simulink model "fusionAlg"  (R2018b)
settings: Solver=FixedStepDiscrete  StartTime=0.0  StopTime=inf  FixedStep=0.01  RelTol=1e-3
PostLoadFcn:
  | if any(exist('dsrtsu_mdlpostloadfcn', 'file') ~= 0), dsrtsu_mdlpostloadfcn('Execute', bdroot); end
model workspace (MAT data in the model file):
  cs : Simulink.ConfigSet (value not decoded)
(part 1 of 24)
settings Model: DSRTSU_INTERNAL_RTI_VER=540  DSRTSU_INTERNAL_RTI_TYPE=rti1401  RTICANMMDATA=struct('GeneralSetupData',struct('modelroot','F:\DatabaseZO\08.Code\Model\ZOP_Integration','generalsettings',struct('filesettings',struct('destfolder',struct('Name','RTICANMM_FILES','Check',1),'buildfolder',struct('Name','.','Check',1),'AbsDestfolder',struct('Name','F:\DatabaseZO\08.Code\Model\ZOP_Integration\RTICANMM_FILES'),'AbsBuildfolder',struct('Name','F:\DatabaseZO\08.Code\Model\ZOP_Integration'))),'options',struct('addpaths',1,'rmpaths',1,'addtrcexclusion',logical(1),'cannavigator',struct('checkmonitoring',0),'show_usrtrc',0,'use_usrtrc',0),'advanced',struct('options',ones(1,100)),'MPSetup',{{}},'RTI',struct('Type','RTI1401','Ver','7.12','Date','02-May-2019'),'modelname','fusionAlg','block','fusionAlg'))  DSRTSU_INTERNAL_RTIFPGA=130  Creator=One-J  LastModifiedBy=zjw
settings OptimizationCC: BlockReduction=off  ConditionallyExecuteInputs=off  DefaultUnderspecifiedDataType=single  BufferReuse=off  EnhancedBackFolding=on  ExpressionFolding=off  PassReuseOutputArgsThreshold=0  LocalBlockOutputs=off  OptimizeBlockOrder=speed  DifferentSizesBufferReuse=on
settings DebuggingCC: ParameterTunabilityLossMsg=error
settings HardwareCC: ProdBitPerPointer=32  ProdBitPerSizeT=32  ProdBitPerPtrDiffT=32  ProdLargestAtomicInteger=Integer  ProdEndianess=BigEndian  ProdWordSize=32  ProdHWDeviceType=Custom Processor->Custom  TargetIntDivRoundTo=Zero  TargetEndianess=BigEndian  TargetHWDeviceType=Custom Processor->Custom
settings ModelReferenceCC: ModelReferenceNumInstancesAllowed=Single
settings SFSimCC: MATLABDynamicMemAlloc=off
settings RTWCC: SystemTargetFile=rti1401.tlc  MakeCommand=make_rti  TemplateMakefile=rti1401.tmf  Description=dSPACE DS1401 Hardware Platform  GenerateReport=on  LaunchReport=on
settings CodeAppCC: OperatorAnnotations=on
settings STFCustomTargetCC: ParMdlRefBuildCompliant=on  SystemTargetFile=rti1401.tlc
settings GRTTargetCC: TargetLangStandard=C89/C90 (ANSI)  CompOptLevelCompliant=off  ConcurrentExecutionCompliant=off  CombineOutputUpdateFcns=off  MatFileLogging=off  CPPClassGenCompliant=off  UseToolchainInfoCompliant=off

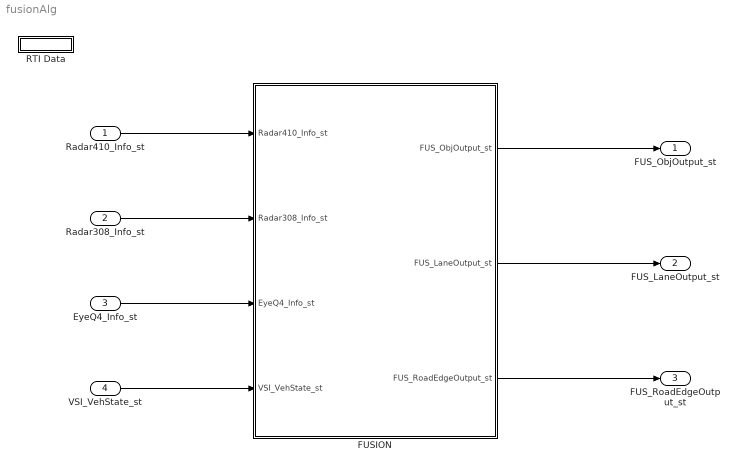
== system fusionAlg ==
  Radar410_Info_st : Inport  OutDataTypeStr=Bus: Radar410_Info_ST
  Radar308_Info_st : Inport  Port=2  OutDataTypeStr=Bus: ARS308_RX  BusOutputAsStruct=on
  EyeQ4_Info_st : Inport  Port=3  OutDataTypeStr=Bus: EYEQ4_DATA_RT_ST  BusOutputAsStruct=on
  VSI_VehState_st : Inport  Port=4  OutDataTypeStr=Bus: VSI_VEHSTATE_ST
  "FUSION " : Subsystem
  RTI Data : Subsystem  Tag=struct('RTIDataServer',struct('RTIDataServerVs','2','RTIModelDescription','struct(''main'',''fusionAlg'',''sub'','''',''isMp'',0)'))  LoadFcn="if exist('rtidc'), try,  rtidc('DataHostBlockClbLoad', gcbh); catch, disp(['Warning: ''LoadFcn'' for RTI Data block failed: ' lasterr]); end, end,"  mask(RTI_DATA_HOST){}
      mask help:
      | RTI Data Block.
      | This block is used by RTI to store internal model-dependent data.
      | Please keep this block on the root level of the model. Deleting this block will result in data loss.
      |
      | NEVER DELETE OR COPY THIS BLOCK!
      settings: CopyFcn="if exist('rtidc'), try,  rtidc('DataHostBlockClbCopy', gcbh); catch, disp(['Warning: ''CopyFcn'' for RTI Data block failed: ' lasterr]); end, end,"  DeleteFcn="if exist('rtidc'), try,  rtidc('DataHostBlockClbDelete', gcbh); catch, disp(['Warning: ''DeleteFcn'' for RTI Data block failed: ' lasterr]); end, end,"  ModelCloseFcn="if exist('rtidc'), try,  rtidc('DataHostBlockClbModelClose', gcbh); catch, disp(['Warning: ''ModelCloseFcn'' for RTI Data block failed: ' lasterr]); end, end,"  PreSaveFcn="if exist('rtidc'), try,  rtidc('DataHostBlockClbPreSave', gcbh); catch, disp(['Warning: ''PreSaveFcn'' for RTI Data block failed: ' lasterr]); end, end,"  PostSaveFcn="if exist('rtidc'), try,  rtidc('DataHostBlockClbPostSave', gcbh); catch, disp(['Warning: ''PostSaveFcn'' for RTI Data block failed: ' lasterr]); end, end,"  NameChangeFcn="if exist('rtidc'), try,  rtidc('DataHostBlockClbNameChange', gcbh); catch, disp(['Warning: ''NameChangeFcn'' for RTI Data block failed: ' lasterr]); end, end,"
      mask Help:
      | RTI Data Block.
      | This block is used by RTI to store internal model-dependent data.
      | Please keep this block on the root level of the model. Deleting this block will result in data loss.
      | 
      | NEVER DELETE OR COPY THIS BLOCK!
      mask Display:
      | text(0.5, 0.5, 'RTI Data', 'HorizontalAlignment', 'center');
      | plot([1 0]);
  "FUS_ObjOutput_st " : Outport  OutDataTypeStr=Bus: FUS_OBJ_OUTPUT_ST  BusOutputAsStruct=on
  FUS_LaneOutput_st : Outport  Port=2  OutDataTypeStr=Bus: FUS_LANE_OUTPUT_ST  BusOutputAsStruct=on
  FUS_RoadEdgeOutput_st : Outport  Port=3  OutDataTypeStr=Bus: FUS_ROAD_EDGE_OUTPUT_ST  BusOutputAsStruct=on
  wires:
  Radar410_Info_st/1 -> "FUSION "/1(Radar410_Info_st)
  EyeQ4_Info_st/1 -> "FUSION "/3(EyeQ4_Info_st)
  "FUSION "/1("FUS_ObjOutput_st ") -> "FUS_ObjOutput_st "/1
  VSI_VehState_st/1 -> "FUSION "/4(VSI_VehState_st)
  "FUSION "/2(FUS_LaneOutput_st) -> FUS_LaneOutput_st/1
  "FUSION "/3(FUS_RoadEdgeOutput_st) -> FUS_RoadEdgeOutput_st/1
  Radar308_Info_st/1 -> "FUSION "/2(Radar308_Info_st)

== system fusionAlg/FUSION  ==
  Radar410_Info_st : Inport  OutDataTypeStr=Bus: Radar410_Info_ST
  Radar308_Info_st : Inport  Port=2  OutDataTypeStr=Bus: ARS308_RX
  EyeQ4_Info_st : Inport  Port=3  OutDataTypeStr=Bus: EYEQ4_DATA_RT_ST
  VSI_VehState_st : Inport  Port=4  OutDataTypeStr=Bus: VSI_VEHSTATE_ST
  FUS_DataAdapter : Subsystem
  FusionAlg : Subsystem
  "FUS_ObjOutput_st " : Outport  OutDataTypeStr=Bus: FUS_OBJ_OUTPUT_ST  BusOutputAsStruct=on
  FUS_LaneOutput_st : Outport  Port=2  OutDataTypeStr=Bus: FUS_LANE_OUTPUT_ST
  FUS_RoadEdgeOutput_st : Outport  Port=3  OutDataTypeStr=Bus: FUS_ROAD_EDGE_OUTPUT_ST
  wires:
  Radar410_Info_st/1 -> FUS_DataAdapter/1(Radar410_Info_st)
  EyeQ4_Info_st/1 -> FUS_DataAdapter/3(EyeQ4_Info_st)
  FusionAlg/1(FUS_ObjOutput_st) -> "FUS_ObjOutput_st "/1  "FUS_ObjOutput_st"
  VSI_VehState_st/1 -> FUS_DataAdapter/4(VSI_VehState_st)
  FUS_DataAdapter/1(FUS_Radar410_st) -> FusionAlg/1(FUS_RadarData_st)  "FUS_Radar410_st"
  FUS_DataAdapter/3(FUS_EgoMotion_st) -> FusionAlg/3(FUS_VehicleData_st)  "FUS_EgoMotion_st"
  FUS_DataAdapter/4(FUS_VisionObjDectection_st) -> FusionAlg/4(FUS_VisionObjData_st)  "FUS_VisObj_st"
  FUS_DataAdapter/5(FUS_VisionLane_st) -> FusionAlg/5(FUS_VisionLaneData_st)  "FUS_VisLane_st"
  FusionAlg/2(FUS_LaneOutput_st) -> FUS_LaneOutput_st/1  "FUS_LaneOutput_st"
  FUS_DataAdapter/6(FUS_RoadEdge_st) -> FusionAlg/6(FUS_RoadEdgeData_st)  "FUS_VisRoadEdge_st"
  FusionAlg/3(FUS_RoadEdgeOutput_st) -> FUS_RoadEdgeOutput_st/1  "FUS_RoadEdgeOutput_st"
  Radar308_Info_st/1 -> FUS_DataAdapter/2(Radar308_Info_st)
  FUS_DataAdapter/2(FUS_Radar308_st) -> FusionAlg/2(FUS_Radar308_st)  "FUS_Radar308_st"

== system fusionAlg/RTI Data ==
  RTI Data Store : Subsystem  Tag="struct('private',struct('version',struct('dsVer',uint32(2),'dsVerCreation',uint32(2),'RTI',struct('ver','7.12','type','RTI1401')),'access',struct('type','Model','isPerm',1,'created',['01-Dec-2020 12:48:00'],'modified',['28-Jan-2021 21:03:50'],'location','')),'public',struct('main',struct('data',[]),'sub',struct('name',{{'fusionAlg'}},'data',{{struct('TH',struct('thTaskInfo',struct('taskType',{'TIMER','HWINT','TMRINT','SWINT','GLINT'},'tasksNumOf',{1,0,0,0,0},'srcIds',{{'TIMERA'},{},{},{},{}},'taskNames',{{['Timer Task 1']},{},{},{},{}})),'th_tc',struct('dataType','TASK','taskGroupId','','taskGroupList',{{}},'taskSchedulingPolicy','FCFS','taskType','TIMER','blkh',-1,'srcId','TIMERA','srcSgnName',['Timer A interrupt'],'srcCpuName','','taskName',['Timer Task 1  [0.005] s'],'taskNameDisplayExt','','smplTime',0.005,'smplTimeOffs',0,'hasFixedPriority',0,'priority',1,'hasFixedOvc',0,'ovcType',1,'ovcMax',1),'tc_th',struct('dataType','TASK','taskGroupId','','taskGroupList',{{}},'taskSchedulingPolicy','FCFS','taskType','TIMER','blkh',-1,'srcId','TIMERA','srcSgnName',['Timer A interrupt'],'srcCpuName','','taskName',['Timer Task 1  [0.005] s'],'taskNameDisplayExt','','smplTime',0.005,'smplTimeOffs',0,'hasFixedPriority',0,'priority',1,'hasFixedOvc',0,'ovcType',1,'ovcMax',1))}})))"  mask(RTI_DATA_STORE){}
      mask help:
      | RTI Data Store Block. This block is used by RTI to store internal model dependent data. Deleting this block will result in data loss.
      |
      | NEVER DELETE, COPY, OR MODIFY THIS BLOCK!
      mask Help:
      | RTI Data Store Block. This block is used by RTI to store internal model dependent data. Deleting this block will result in data loss.
      | 
      | NEVER DELETE, COPY, OR MODIFY THIS BLOCK!
      mask Display: text(0.5, 0.5, ' ', 'HorizontalAlignment', 'center');

== system fusionAlg/FUSION /FUS_DataAdapter ==
  Radar410_Info_st : Inport  OutDataTypeStr=Bus: Radar410_Info_ST
  Radar308_Info_st : Inport  Port=2  OutDataTypeStr=Bus: ARS308_RX
  EyeQ4_Info_st : Inport  Port=3  OutDataTypeStr=Bus: EYEQ4_DATA_RT_ST
  VSI_VehState_st : Inport  Port=4  OutDataTypeStr=Bus: VSI_VEHSTATE_ST
  ARS308Adapter : Subsystem
  EgoMotionAdapter : Subsystem
  RadarAdapter : Subsystem
  VisionAdapter : Subsystem
  FUS_Radar410_st : Outport  OutDataTypeStr=Bus: FUS_RADAR_DATA_ST
  FUS_Radar308_st : Outport  Port=2  OutDataTypeStr=Bus: FUS_ARS308_DATA_ST
  FUS_EgoMotion_st : Outport  Port=3  OutDataTypeStr=Bus: FUS_VEHICLE_DATA_ST
  FUS_VisionObjDectection_st : Outport  Port=4  OutDataTypeStr=Bus: FUS_VISION_OBJ_DATA_ST
  FUS_VisionLane_st : Outport  Port=5  OutDataTypeStr=Bus: FUS_EYEQ4_LANE_DATA_ST
  FUS_RoadEdge_st : Outport  Port=6  OutDataTypeStr=Bus: FUS_EYEQ4_ROADEDGE_DATA_ST
  wires:
  Radar410_Info_st/1 -> RadarAdapter/1(Radar410_Info_st)
  RadarAdapter/1(FUS_Radar410_st) -> FUS_Radar410_st/1
  VisionAdapter/1(FUS_Vision_OD_st) -> FUS_VisionObjDectection_st/1
  EyeQ4_Info_st/1 -> VisionAdapter/1(In_VisionData)
  VSI_VehState_st/1 -> EgoMotionAdapter/1(VSI_VehState_st)
  EgoMotionAdapter/1(FUS_EgoMotion_st) -> FUS_EgoMotion_st/1
  VisionAdapter/2(FUS_Vision_Lane_st) -> FUS_VisionLane_st/1
  Radar308_Info_st/1 -> ARS308Adapter/1(Radar308_Info_st)
  ARS308Adapter/1(FUS_Radar308_st) -> FUS_Radar308_st/1
  VisionAdapter/3(FUS_Vision_RoadEdge_st) -> FUS_RoadEdge_st/1

== system fusionAlg/FUSION /FusionAlg ==
  FUS_RadarData_st : Inport  OutDataTypeStr=Bus: FUS_RADAR_DATA_ST
  FUS_Radar308_st : Inport  Port=2  OutDataTypeStr=Bus: FUS_ARS308_DATA_ST
  FUS_VehicleData_st : Inport  Port=3  OutDataTypeStr=Bus: FUS_VEHICLE_DATA_ST
  FUS_VisionObjData_st : Inport  Port=4  OutDataTypeStr=Bus: FUS_VISION_OBJ_DATA_ST
  FUS_VisionLaneData_st : Inport  Port=5  OutDataTypeStr=Bus: FUS_EYEQ4_LANE_DATA_ST
  FUS_RoadEdgeData_st : Inport  Port=6  OutDataTypeStr=Bus: FUS_EYEQ4_ROADEDGE_DATA_ST
  BusToBusArray : Subsystem
  Constant : Constant  Value=0  OutDataTypeStr=uint16
  FusionAlg : S-Function  InitFcn=try, set_param(gcb,'FunctionName','funsionAlg_sfun'), end  FunctionName=funsionAlg_sfun  SFunctionModules=funsionAlg_sfun_wrapper fusion_process sensor_adapter coordinate_align double_bounce_remover signal_preprocess datastruct_fusion_internal_state fusion_predict radar_track_predict predict association cluster_update group splitter fusion_track_manager fusion_update track_manager post_fusion_process output_adapter combine_all_radar  SFunctionDeploymentMode=off  EnableBusSupport=off  mask(S-Function Builder){}
      mask help: Simulink:masks:SFunctionBuilder_MD
      mask init:
      | val = [[.9  0.75 0.75 1 1 .9 .9 1]',[1 1 0.75 0.75 .9 .9 1 .9]'];try , sys = get_param(gcb,'SfunBuilderFcnName');if isempty(sys), sys = get_param(gcb,'FunctionName'); end,catch, sys = get_param(gcb,'FunctionName'); end
      settings: CopyFcn=set_param(gcbh,'LinkStatus','none')  PreSaveFcn=try, set_param(gcb,'FunctionName','funsionAlg_sfun'), end  OpenFcn=sfunctionwizard(gcbh)
      mask Display: plot(val(:,1),val(:,2)),disp(sys), port_label('input',1,'In_RadarData_st'), port_label('input',2,'In_ARS308Data_st'), port_label('input',3,'In_VehicleData_st'), port_label('input',4,'In_VisionObjData_st'), port_label('input',5,'In_VisionLaneData_st'), port_label('input',6,'In_VisionRoadEdgeData_st'), port_label('input',7,'In_ErrorFlag'), port_label('output',1,'Out_FusionObjInfo_st'), port_label('output',2,'Out_FusionLaneInfo_st'), port_label('output',3,'Out_FusionRoadEdgeInfo_st')
  FUS_ObjOutput_st : Outport  OutDataTypeStr=Bus: FUS_OBJ_OUTPUT_ST
  FUS_LaneOutput_st : Outport  Port=2  OutDataTypeStr=Bus: FUS_LANE_OUTPUT_ST
  FUS_RoadEdgeOutput_st : Outport  Port=3  OutDataTypeStr=Bus: FUS_ROAD_EDGE_OUTPUT_ST
  wires:
  FUS_RadarData_st/1 -> FusionAlg/1
  FUS_VehicleData_st/1 -> FusionAlg/3
  FUS_VisionObjData_st/1 -> FusionAlg/4
  FUS_VisionLaneData_st/1 -> FusionAlg/5
  FUS_RoadEdgeData_st/1 -> FusionAlg/6
  FusionAlg/2 -> FUS_LaneOutput_st/1
  FusionAlg/1 -> BusToBusArray/1(Out_FusionObjInfo_st)
  BusToBusArray/1(FUS_ObjOutput_st) -> FUS_ObjOutput_st/1
  FusionAlg/3 -> FUS_RoadEdgeOutput_st/1
  FUS_Radar308_st/1 -> FusionAlg/2
  Constant/1 -> FusionAlg/7

== system fusionAlg/RTI Data/RTI Data Store ==
  RTI Data Store : Subsystem  mask(RTI_DATA_STORE){}
      mask help:
      | RTI Data Store Block. This block is used by RTI to store internal model dependent data. Deleting this block will result in data loss.
      |
      | NEVER DELETE, COPY, OR MODIFY THIS BLOCK!
      mask Help:
      | RTI Data Store Block. This block is used by RTI to store internal model dependent data. Deleting this block will result in data loss.
      | 
      | NEVER DELETE, COPY, OR MODIFY THIS BLOCK!
      mask Display: text(0.5, 0.5, ' ', 'HorizontalAlignment', 'center');

== system fusionAlg/FUSION /FUS_DataAdapter/ARS308Adapter ==
  Radar308_Info_st : Inport
  Bus Creator : BusCreator  Inputs=4  OutDataTypeStr=Bus: FUS_ARS308_DATA_ST  NonVirtualBus=on
      settings: InheritFromInputs=off
  Bus Selector : BusSelector  OutputSignals=leftFrontRadar_General,LeftFrontRadar_Status,rightFrontRadar_General,rightFrontRadar_Status,rightRearRadar_General,rightRearRadar_Status,leftRearRadar_General,leftRearRadar_Status
  leftFrontRadar : Subsystem
  leftRearRadar : Subsystem
  rightFrontRadar : Subsystem
  rightRearRadar : Subsystem
  FUS_Radar308_st : Outport
  wires:
  Bus Creator/1 -> FUS_Radar308_st/1
  Radar308_Info_st/1 -> Bus Selector/1
  Bus Selector/1 -> leftFrontRadar/1(<leftRearRadar_General>)  "<leftFrontRadar_General>"
  leftFrontRadar/1(FUS_Radar410_st) -> Bus Creator/1  "leftFrontRadar"
  rightFrontRadar/1(FUS_Radar410_st) -> Bus Creator/2  "rightFrontRadar"
  rightRearRadar/1(FUS_Radar410_st) -> Bus Creator/3  "rightRearRadar"
  leftRearRadar/1(FUS_Radar410_st) -> Bus Creator/4  "leftRearRadar"
  Bus Selector/2 -> leftFrontRadar/2(<leftRearRadar_Status>)  "<LeftFrontRadar_Status>"
  Bus Selector/3 -> rightFrontRadar/1(<rightFrontRadar_General>)  "<rightFrontRadar_General>"
  Bus Selector/4 -> rightFrontRadar/2(<rightFrontRadar_Status>)  "<rightFrontRadar_Status>"
  Bus Selector/5 -> rightRearRadar/1(<rightRearRadar_General>)  "<rightRearRadar_General>"
  Bus Selector/6 -> rightRearRadar/2(<rightRearRadar_Status>)  "<rightRearRadar_Status>"
  Bus Selector/7 -> leftRearRadar/1(<leftRearRadar_General>)  "<leftRearRadar_General>"
  Bus Selector/8 -> leftRearRadar/2(<leftRearRadar_Status>)  "<leftRearRadar_Status>"

== system fusionAlg/FUSION /FUS_DataAdapter/EgoMotionAdapter ==
  VSI_VehState_st : Inport  OutDataTypeStr=Bus: VSI_VEHSTATE_ST
  Bus Creator : BusCreator  Inputs=4  OutDataTypeStr=Bus: FUS_VEHICLE_DATA_ST  NonVirtualBus=on
      settings: InheritFromInputs=off
  Bus Selector : BusSelector  OutputSignals=YrsF,vRef,aRef
  motionStatus : Constant  OutDataTypeStr=single
  FUS_EgoMotion_st : Outport
  wires:
  VSI_VehState_st/1 -> Bus Selector/1
  Bus Creator/1 -> FUS_EgoMotion_st/1
  motionStatus/1 -> Bus Creator/2  "MotionStatus"
  Bus Selector/1 -> Bus Creator/1  "<YrsF>"
  Bus Selector/2 -> Bus Creator/3  "<vRef>"
  Bus Selector/3 -> Bus Creator/4  "<aRef>"

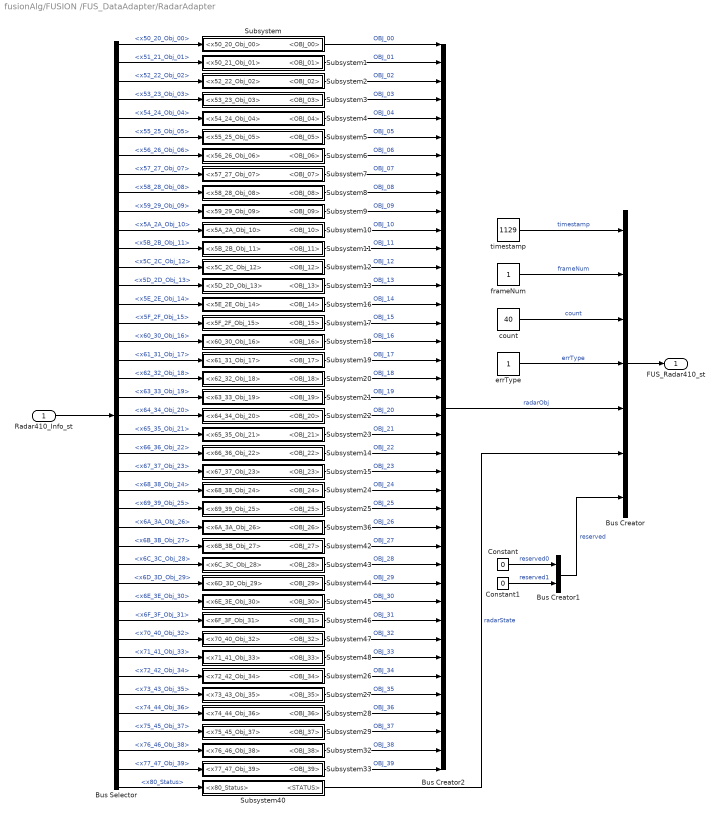
== system fusionAlg/FUSION /FUS_DataAdapter/RadarAdapter ==
  Radar410_Info_st : Inport
  Bus Creator : BusCreator  Inputs=7  OutDataTypeStr=Bus: FUS_RADAR_DATA_ST  NonVirtualBus=on
      settings: InheritFromInputs=off
  Bus Creator1 : BusCreator  Inputs=2  OutDataTypeStr=Bus: FUS_UINT32_RESERVED_ST  NonVirtualBus=on
      settings: InheritFromInputs=off
  Bus Creator2 : BusCreator  Inputs=40  OutDataTypeStr=Bus: FUS_RADOBJ_LIST_ST  NonVirtualBus=on
      settings: InheritFromInputs=off
  Bus Selector : BusSelector  OutputSignals=x50_20_Obj_00,x51_21_Obj_01,x52_22_Obj_02,x53_23_Obj_03,x54_24_Obj_04,x55_25_Obj_05,x56_26_Obj_06,x57_27_Obj_07,x58_28_Obj_08,x59_29_Obj_09,x5A_2A_Obj_10,x5B_2B_Obj_11,x5C_2C_Obj_12,x5D_2D_Obj_13,x5E_2E_Obj_14,x5F_2F_Obj_15,x60_30_Obj_16,x61_31_Obj_17,x62_32_Obj_18,x63_33_Obj_19,x64_34_Obj_20,x65_35_Obj_21,x66_36_Obj_22,x67_37_Obj_23,x68_38_Obj_24,x69_39_Obj_25,x6A_3A_Obj_26,x6B_3B_Obj_27,x6C_3C_Obj_28,x6D_3D_Obj_29,x6E_3E_Obj_30,x6F_3F_Obj_31,x70_40_Obj_32,x71_41_Obj_33,x72_42_Obj_34,x73_43_Obj_35,x74_44_Obj_36,x75_45_Obj_37,x76_46_Obj_38,x77_47_Obj_39,x80_Status
  Constant : Constant  Value=0  OutDataTypeStr=uint32
  Constant1 : Constant  Value=0  OutDataTypeStr=uint32
  Subsystem : Subsystem
  Subsystem1 : Subsystem
  Subsystem10 : Subsystem
  Subsystem11 : Subsystem
  Subsystem12 : Subsystem
  Subsystem13 : Subsystem
  Subsystem14 : Subsystem
  Subsystem15 : Subsystem
  Subsystem16 : Subsystem
  Subsystem17 : Subsystem
  Subsystem18 : Subsystem
  Subsystem19 : Subsystem
  Subsystem2 : Subsystem
  Subsystem20 : Subsystem
  Subsystem21 : Subsystem
  Subsystem22 : Subsystem
  Subsystem23 : Subsystem
  Subsystem24 : Subsystem
  Subsystem25 : Subsystem
  Subsystem26 : Subsystem
  Subsystem27 : Subsystem
  Subsystem28 : Subsystem
  Subsystem29 : Subsystem
  Subsystem3 : Subsystem
  Subsystem32 : Subsystem
  Subsystem33 : Subsystem
  Subsystem36 : Subsystem
  Subsystem4 : Subsystem
  Subsystem40 : Subsystem
  Subsystem42 : Subsystem
  Subsystem43 : Subsystem
  Subsystem44 : Subsystem
  Subsystem45 : Subsystem
  Subsystem46 : Subsystem
  Subsystem47 : Subsystem
  Subsystem48 : Subsystem
  Subsystem5 : Subsystem
  Subsystem6 : Subsystem
  Subsystem7 : Subsystem
  Subsystem8 : Subsystem
  Subsystem9 : Subsystem
  count : Constant  Value=40  OutDataTypeStr=uint32
  errType : Constant  OutDataTypeStr=uint32
  frameNum : Constant  OutDataTypeStr=uint32
  timestamp : Constant  Value=1129
  FUS_Radar410_st : Outport  OutDataTypeStr=Bus: FUS_RADAR_DATA_ST
  wires:
  Radar410_Info_st/1 -> Bus Selector/1
  Bus Creator/1 -> FUS_Radar410_st/1
  Bus Selector/1 -> Subsystem/1(<x50_20_Obj_00>)  "<x50_20_Obj_00>"
  Bus Selector/2 -> Subsystem1/1(<x50_21_Obj_01>)  "<x51_21_Obj_01>"
  Bus Selector/3 -> Subsystem2/1(<x52_22_Obj_02>)  "<x52_22_Obj_02>"
  Bus Selector/41 -> Subsystem40/1(<x80_Status>)  "<x80_Status>"
  Subsystem/1(<OBJ_00>) -> Bus Creator2/1  "OBJ_00"
  Subsystem1/1(<OBJ_01>) -> Bus Creator2/2  "OBJ_01"
  timestamp/1 -> Bus Creator/1  "timestamp"
  frameNum/1 -> Bus Creator/2  "frameNum"
  count/1 -> Bus Creator/3  "count"
  Bus Creator2/1 -> Bus Creator/5  "radarObj"
  Subsystem40/1(<STATUS>) -> Bus Creator/6  "radarState"
  Constant1/1 -> Bus Creator1/2  "reserved1"
  Constant/1 -> Bus Creator1/1  "reserved0"
  Bus Creator1/1 -> Bus Creator/7  "reserved"
  Subsystem2/1(<OBJ_02>) -> Bus Creator2/3  "OBJ_02"
  Subsystem5/1(<OBJ_05>) -> Bus Creator2/6  "OBJ_05"
  Bus Selector/6 -> Subsystem5/1(<x55_25_Obj_05>)  "<x55_25_Obj_05>"
  Subsystem3/1(<OBJ_03>) -> Bus Creator2/4  "OBJ_03"
  Bus Selector/4 -> Subsystem3/1(<x53_23_Obj_03>)  "<x53_23_Obj_03>"
  Subsystem4/1(<OBJ_04>) -> Bus Creator2/5  "OBJ_04"
  Bus Selector/5 -> Subsystem4/1(<x54_24_Obj_04>)  "<x54_24_Obj_04>"
  Bus Selector/9 -> Subsystem8/1(<x58_28_Obj_08>)  "<x58_28_Obj_08>"
  Bus Selector/11 -> Subsystem10/1(<x5A_2A_Obj_10>)  "<x5A_2A_Obj_10>"
  Subsystem9/1(<OBJ_09>) -> Bus Creator2/10  "OBJ_09"
  Bus Selector/12 -> Subsystem11/1(<x5B_2B_Obj_11>)  "<x5B_2B_Obj_11>"
  Subsystem11/1(<OBJ_11>) -> Bus Creator2/12  "OBJ_11"
  Subsystem8/1(<OBJ_08>) -> Bus Creator2/9  "OBJ_08"
  Subsystem6/1(<OBJ_06>) -> Bus Creator2/7  "OBJ_06"
  Bus Selector/7 -> Subsystem6/1(<x56_26_Obj_06>)  "<x56_26_Obj_06>"
  Subsystem7/1(<OBJ_07>) -> Bus Creator2/8  "OBJ_07"
  Bus Selector/8 -> Subsystem7/1(<x57_27_Obj_07>)  "<x57_27_Obj_07>"
  Bus Selector/10 -> Subsystem9/1(<x59_29_Obj_09>)  "<x59_29_Obj_09>"
  Subsystem10/1(<OBJ_10>) -> Bus Creator2/11  "OBJ_10"
  Subsystem14/1(<OBJ_22>) -> Bus Creator2/23  "OBJ_22"
  Bus Selector/19 -> Subsystem20/1(<x62_32_Obj_18>)  "<x62_32_Obj_18>"
  Bus Selector/22 -> Subsystem23/1(<x65_35_Obj_21>)  "<x65_35_Obj_21>"
  Bus Selector/24 -> Subsystem15/1(<x67_37_Obj_23>)  "<x67_37_Obj_23>"
  Subsystem22/1(<OBJ_20>) -> Bus Creator2/21  "OBJ_20"
  Subsystem15/1(<OBJ_23>) -> Bus Creator2/24  "OBJ_23"
  Subsystem20/1(<OBJ_18>) -> Bus Creator2/19  "OBJ_18"
  Subsystem21/1(<OBJ_19>) -> Bus Creator2/20  "OBJ_19"
  Subsystem23/1(<OBJ_21>) -> Bus Creator2/22  "OBJ_21"
  Bus Selector/21 -> Subsystem22/1(<x64_34_Obj_20>)  "<x64_34_Obj_20>"
  Bus Selector/15 -> Subsystem16/1(<x5E_2E_Obj_14>)  "<x5E_2E_Obj_14>"
  Bus Selector/23 -> Subsystem14/1(<x66_36_Obj_22>)  "<x66_36_Obj_22>"
  Bus Selector/17 -> Subsystem18/1(<x60_30_Obj_16>)  "<x60_30_Obj_16>"
  Subsystem17/1(<OBJ_15>) -> Bus Creator2/16  "OBJ_15"
  Bus Selector/18 -> Subsystem19/1(<x61_31_Obj_17>)  "<x61_31_Obj_17>"
  Subsystem12/1(<OBJ_12>) -> Bus Creator2/13  "OBJ_12"
  Bus Selector/13 -> Subsystem12/1(<x5C_2C_Obj_12>)  "<x5C_2C_Obj_12>"
  Subsystem13/1(<OBJ_13>) -> Bus Creator2/14  "OBJ_13"
  Bus Selector/14 -> Subsystem13/1(<x5D_2D_Obj_13>)  "<x5D_2D_Obj_13>"
  Subsystem18/1(<OBJ_16>) -> Bus Creator2/17  "OBJ_16"
  Bus Selector/16 -> Subsystem17/1(<x5F_2F_Obj_15>)  "<x5F_2F_Obj_15>"
  Bus Selector/20 -> Subsystem21/1(<x63_33_Obj_19>)  "<x63_33_Obj_19>"
  Subsystem19/1(<OBJ_17>) -> Bus Creator2/18  "OBJ_17"
  Subsystem16/1(<OBJ_14>) -> Bus Creator2/15  "OBJ_14"
  Subsystem26/1(<OBJ_34>) -> Bus Creator2/35  "OBJ_34"
  Bus Selector/31 -> Subsystem45/1(<x6E_3E_Obj_30>)  "<x6E_3E_Obj_30>"
  Bus Selector/34 -> Subsystem48/1(<x71_41_Obj_33>)  "<x71_41_Obj_33>"
  Bus Selector/36 -> Subsystem27/1(<x73_43_Obj_35>)  "<x73_43_Obj_35>"
  Subsystem27/1(<OBJ_35>) -> Bus Creator2/36  "OBJ_35"
  Subsystem45/1(<OBJ_30>) -> Bus Creator2/31  "OBJ_30"
  Subsystem46/1(<OBJ_31>) -> Bus Creator2/32  "OBJ_31"
  Subsystem48/1(<OBJ_33>) -> Bus Creator2/34  "OBJ_33"
  Bus Selector/40 -> Subsystem33/1(<x77_47_Obj_39>)  "<x77_47_Obj_39>"
  Bus Selector/33 -> Subsystem47/1(<x70_40_Obj_32>)  "<x70_40_Obj_32>"
  Bus Selector/27 -> Subsystem36/1(<x6A_3A_Obj_26>)  "<x6A_3A_Obj_26>"
  Bus Selector/35 -> Subsystem26/1(<x72_42_Obj_34>)  "<x72_42_Obj_34>"
  Bus Selector/29 -> Subsystem43/1(<x6C_3C_Obj_28>)  "<x6C_3C_Obj_28>"
  Bus Selector/30 -> Subsystem44/1(<x6D_3D_Obj_29>)  "<x6D_3D_Obj_29>"
  Subsystem42/1(<OBJ_27>) -> Bus Creator2/28  "OBJ_27"
  Subsystem28/1(<OBJ_36>) -> Bus Creator2/37  "OBJ_36"
  Subsystem29/1(<OBJ_37>) -> Bus Creator2/38  "OBJ_37"
  Bus Selector/39 -> Subsystem32/1(<x76_46_Obj_38>)  "<x76_46_Obj_38>"
  Subsystem24/1(<OBJ_24>) -> Bus Creator2/25  "OBJ_24"
  Subsystem32/1(<OBJ_38>) -> Bus Creator2/39  "OBJ_38"
  Subsystem43/1(<OBJ_28>) -> Bus Creator2/29  "OBJ_28"
  Bus Selector/28 -> Subsystem42/1(<x6B_3B_Obj_27>)  "<x6B_3B_Obj_27>"
  Bus Selector/38 -> Subsystem29/1(<x75_45_Obj_37>)  "<x75_45_Obj_37>"
  Subsystem33/1(<OBJ_39>) -> Bus Creator2/40  "OBJ_39"
  Bus Selector/25 -> Subsystem24/1(<x68_38_Obj_24>)  "<x68_38_Obj_24>"
  Subsystem47/1(<OBJ_32>) -> Bus Creator2/33  "OBJ_32"
  Bus Selector/37 -> Subsystem28/1(<x74_44_Obj_36>)  "<x74_44_Obj_36>"
  Subsystem25/1(<OBJ_25>) -> Bus Creator2/26  "OBJ_25"
  Bus Selector/26 -> Subsystem25/1(<x69_39_Obj_25>)  "<x69_39_Obj_25>"
  Bus Selector/32 -> Subsystem46/1(<x6F_3F_Obj_31>)  "<x6F_3F_Obj_31>"
  Subsystem44/1(<OBJ_29>) -> Bus Creator2/30  "OBJ_29"
  Subsystem36/1(<OBJ_26>) -> Bus Creator2/27  "OBJ_26"
  errType/1 -> Bus Creator/4  "errType"

== system fusionAlg/FUSION /FUS_DataAdapter/VisionAdapter ==
  In_VisionData : Inport  OutDataTypeStr=Bus: EYEQ4_DATA_RT_ST
  Bus Selector : BusSelector  OutputSignals=OBJ_BUS,OBJ_FRAME_INFO,LANE_DATA_ST,ROADEDGE_ST
  LaneAdapter : Subsystem
  ObjAdapter : Subsystem
  RoadEdgeAdapter : Subsystem
  FUS_Vision_OD_st : Outport  OutDataTypeStr=Bus: FUS_VISION_OBJ_DATA_ST
  FUS_Vision_Lane_st : Outport  Port=2  OutDataTypeStr=Bus: FUS_EYEQ4_LANE_DATA_ST
  FUS_Vision_RoadEdge_st : Outport  Port=3  OutDataTypeStr=Bus: FUS_EYEQ4_ROADEDGE_DATA_ST
  wires:
  In_VisionData/1 -> Bus Selector/1
  Bus Selector/3 -> LaneAdapter/1(<LANE_DATA_ST>)  "<LANE_DATA_ST>"
  LaneAdapter/1(FUS_Vision_Lane_st) -> FUS_Vision_Lane_st/1
  Bus Selector/1 -> ObjAdapter/1(OBJ_BUS)  "<OBJ_BUS>"
  ObjAdapter/1(FUS_Vision_OD_st) -> FUS_Vision_OD_st/1
  Bus Selector/2 -> ObjAdapter/2(Obj_Frame_Info)  "<OBJ_FRAME_INFO>"
  Bus Selector/4 -> RoadEdgeAdapter/1(<ROADEDGE_ST>)  "<ROADEDGE_ST>"
  RoadEdgeAdapter/1(FUS_RoadEdge_st) -> FUS_Vision_RoadEdge_st/1

== system fusionAlg/FUSION /FusionAlg/BusToBusArray ==
  Out_FusionObjInfo_st : Inport
  Bus Creator : BusCreator  Inputs=3  OutDataTypeStr=Bus: FUS_OBJ_OUTPUT_ST  NonVirtualBus=on
  Bus Selector : BusSelector  OutputSignals=timeStamp,objects,frameNum
  BusToBusArray : Subsystem
  FUS_ObjOutput_st : Outport
  wires:
  Bus Selector/1 -> Bus Creator/1  "<timeStamp>"
  Bus Creator/1 -> FUS_ObjOutput_st/1
  BusToBusArray/1(BusArray) -> Bus Creator/2  "objects"
  Bus Selector/2 -> BusToBusArray/1(N_Bus)  "<objects>"
  Bus Selector/3 -> Bus Creator/3  "<frameNum>"
  Out_FusionObjInfo_st/1 -> Bus Selector/1

== system fusionAlg/RTI Data/RTI Data Store/RTI Data Store ==
  RTI Data Store : Subsystem  mask(RTI_DATA_STORE){}
      mask help:
      | RTI Data Store Block. This block is used by RTI to store internal model dependent data. Deleting this block will result in data loss.
      |
      | NEVER DELETE, COPY, OR MODIFY THIS BLOCK!
      mask Help:
      | RTI Data Store Block. This block is used by RTI to store internal model dependent data. Deleting this block will result in data loss.
      | 
      | NEVER DELETE, COPY, OR MODIFY THIS BLOCK!
      mask Display: text(0.5, 0.5, ' ', 'HorizontalAlignment', 'center');

== system fusionAlg/FUSION /FUS_DataAdapter/ARS308Adapter/leftFrontRadar ==
  <leftRearRadar_General> : Inport
  <leftRearRadar_Status> : Inport  Port=2
  Bus Creator : BusCreator  Inputs=7  OutDataTypeStr=Bus: FUS_RADAR_DATA_ST  NonVirtualBus=on
      settings: InheritFromInputs=off
  Bus Creator1 : BusCreator  Inputs=2  OutDataTypeStr=Bus: FUS_UINT32_RESERVED_ST  NonVirtualBus=on
      settings: InheritFromInputs=off
  Bus Selector : BusSelector  OutputSignals=tStamp,ObjNum,Version
  Constant : Constant  Value=0  OutDataTypeStr=uint32
  Constant1 : Constant  Value=0  OutDataTypeStr=uint32
  Data Type Conversion : DataTypeConversion  OutDataTypeStr=uint32
  Data Type Conversion1 : DataTypeConversion  OutDataTypeStr=uint32
  Subsystem1 : Subsystem
  Subsystem40 : Subsystem
  errType : Constant  OutDataTypeStr=uint32
  timestamp : Constant  Value=1110
  FUS_Radar410_st : Outport  OutDataTypeStr=Bus: FUS_RADAR_DATA_ST
  wires:
  <leftRearRadar_General>/1 -> Subsystem1/1(<stateHeader>)
  timestamp/1 -> Bus Creator/1  "timestamp"
  errType/1 -> Bus Creator/4  "errType"
  Constant/1 -> Bus Creator1/1  "reserved0"
  Bus Creator/1 -> FUS_Radar410_st/1
  Bus Creator1/1 -> Bus Creator/7  "reserved"
  Constant1/1 -> Bus Creator1/2  "reserved1"
  Subsystem1/1(ARS308Obj) -> Bus Creator/5
  <leftRearRadar_Status>/1 -> Bus Selector/1
  Bus Selector/1 -> Subsystem40/1(<MeasCounter>)  "<tStamp>"
  Bus Selector/2 -> Data Type Conversion/1  "<ObjNum>"
  Bus Selector/3 -> Data Type Conversion1/1  "<Version>"
  Data Type Conversion/1 -> Bus Creator/3  "Count"
  Data Type Conversion1/1 -> Bus Creator/2  "frameNum"
  Subsystem40/1(<STATUS>) -> Bus Creator/6  "radarState"

== system fusionAlg/FUSION /FUS_DataAdapter/ARS308Adapter/leftRearRadar ==
  <leftRearRadar_General> : Inport
  <leftRearRadar_Status> : Inport  Port=2
  Bus Creator : BusCreator  Inputs=7  OutDataTypeStr=Bus: FUS_RADAR_DATA_ST  NonVirtualBus=on
      settings: InheritFromInputs=off
  Bus Creator1 : BusCreator  Inputs=2  OutDataTypeStr=Bus: FUS_UINT32_RESERVED_ST  NonVirtualBus=on
      settings: InheritFromInputs=off
  Bus Selector : BusSelector  OutputSignals=tStamp,ObjNum,Version
  Constant : Constant  Value=0  OutDataTypeStr=uint32
  Constant1 : Constant  Value=0  OutDataTypeStr=uint32
  Data Type Conversion : DataTypeConversion  OutDataTypeStr=uint32
  Data Type Conversion1 : DataTypeConversion  OutDataTypeStr=uint32
  Subsystem1 : Subsystem
  Subsystem40 : Subsystem
  errType : Constant  OutDataTypeStr=uint32
  timestamp : Constant  Value=1116
  FUS_Radar410_st : Outport  OutDataTypeStr=Bus: FUS_RADAR_DATA_ST
  wires:
  <leftRearRadar_General>/1 -> Subsystem1/1(<stateHeader>)
  timestamp/1 -> Bus Creator/1  "timestamp"
  errType/1 -> Bus Creator/4  "errType"
  Constant/1 -> Bus Creator1/1  "reserved0"
  Bus Creator/1 -> FUS_Radar410_st/1
  Bus Creator1/1 -> Bus Creator/7  "reserved"
  Constant1/1 -> Bus Creator1/2  "reserved1"
  Subsystem1/1(ARS308Obj) -> Bus Creator/5
  <leftRearRadar_Status>/1 -> Bus Selector/1
  Bus Selector/1 -> Subsystem40/1(<MeasCounter>)  "<tStamp>"
  Bus Selector/2 -> Data Type Conversion/1  "<ObjNum>"
  Bus Selector/3 -> Data Type Conversion1/1  "<Version>"
  Data Type Conversion/1 -> Bus Creator/3  "Count"
  Data Type Conversion1/1 -> Bus Creator/2  "frameNum"
  Subsystem40/1(<STATUS>) -> Bus Creator/6  "radarState"

== system fusionAlg/FUSION /FUS_DataAdapter/ARS308Adapter/rightFrontRadar ==
  <rightFrontRadar_General> : Inport
  <rightFrontRadar_Status> : Inport  Port=2
  Bus Creator : BusCreator  Inputs=7  OutDataTypeStr=Bus: FUS_RADAR_DATA_ST  NonVirtualBus=on
      settings: InheritFromInputs=off
  Bus Creator1 : BusCreator  Inputs=2  OutDataTypeStr=Bus: FUS_UINT32_RESERVED_ST  NonVirtualBus=on
      settings: InheritFromInputs=off
  Bus Selector : BusSelector  OutputSignals=tStamp,ObjNum,Version
  Constant : Constant  Value=0  OutDataTypeStr=uint32
  Constant1 : Constant  Value=0  OutDataTypeStr=uint32
  Data Type Conversion : DataTypeConversion  OutDataTypeStr=uint32
  Data Type Conversion1 : DataTypeConversion  OutDataTypeStr=uint32
  Subsystem1 : Subsystem
  Subsystem40 : Subsystem
  errType : Constant  OutDataTypeStr=uint32
  timestamp : Constant  Value=1116
  FUS_Radar410_st : Outport  OutDataTypeStr=Bus: FUS_RADAR_DATA_ST
  wires:
  <rightFrontRadar_General>/1 -> Subsystem1/1(<stateHeader>)
  timestamp/1 -> Bus Creator/1  "timestamp"
  errType/1 -> Bus Creator/4  "errType"
  Constant/1 -> Bus Creator1/1  "reserved0"
  Bus Creator/1 -> FUS_Radar410_st/1
  Bus Creator1/1 -> Bus Creator/7  "reserved"
  Constant1/1 -> Bus Creator1/2  "reserved1"
  Subsystem1/1(ARS308Obj) -> Bus Creator/5
  <rightFrontRadar_Status>/1 -> Bus Selector/1
  Bus Selector/1 -> Subsystem40/1(<MeasCounter>)  "<tStamp>"
  Bus Selector/2 -> Data Type Conversion/1  "<ObjNum>"
  Bus Selector/3 -> Data Type Conversion1/1  "<Version>"
  Data Type Conversion/1 -> Bus Creator/3  "Count"
  Data Type Conversion1/1 -> Bus Creator/2  "frameNum"
  Subsystem40/1(<STATUS>) -> Bus Creator/6  "radarState"

== system fusionAlg/FUSION /FUS_DataAdapter/ARS308Adapter/rightRearRadar ==
  <rightRearRadar_General> : Inport
  <rightRearRadar_Status> : Inport  Port=2
  Bus Creator : BusCreator  Inputs=7  OutDataTypeStr=Bus: FUS_RADAR_DATA_ST  NonVirtualBus=on
      settings: InheritFromInputs=off
  Bus Creator1 : BusCreator  Inputs=2  OutDataTypeStr=Bus: FUS_UINT32_RESERVED_ST  NonVirtualBus=on
      settings: InheritFromInputs=off
  Bus Selector : BusSelector  OutputSignals=tStamp,ObjNum,Version
  Constant : Constant  Value=0  OutDataTypeStr=uint32
  Constant1 : Constant  Value=0  OutDataTypeStr=uint32
  Data Type Conversion : DataTypeConversion  OutDataTypeStr=uint32
  Data Type Conversion1 : DataTypeConversion  OutDataTypeStr=uint32
  Subsystem1 : Subsystem
  Subsystem40 : Subsystem
  errType : Constant  OutDataTypeStr=uint32
  timestamp : Constant  Value=1116
  FUS_Radar410_st : Outport  OutDataTypeStr=Bus: FUS_RADAR_DATA_ST
  wires:
  <rightRearRadar_General>/1 -> Subsystem1/1(<stateHeader>)
  timestamp/1 -> Bus Creator/1  "timestamp"
  errType/1 -> Bus Creator/4  "errType"
  Constant/1 -> Bus Creator1/1  "reserved0"
  Bus Creator/1 -> FUS_Radar410_st/1
  Bus Creator1/1 -> Bus Creator/7  "reserved"
  Constant1/1 -> Bus Creator1/2  "reserved1"
  Subsystem1/1(ARS308Obj) -> Bus Creator/5
  <rightRearRadar_Status>/1 -> Bus Selector/1
  Bus Selector/1 -> Subsystem40/1(<MeasCounter>)  "<tStamp>"
  Bus Selector/2 -> Data Type Conversion/1  "<ObjNum>"
  Bus Selector/3 -> Data Type Conversion1/1  "<Version>"
  Data Type Conversion/1 -> Bus Creator/3  "Count"
  Data Type Conversion1/1 -> Bus Creator/2  "frameNum"
  Subsystem40/1(<STATUS>) -> Bus Creator/6  "radarState"

== system fusionAlg/FUSION /FUS_DataAdapter/RadarAdapter/Subsystem ==
  <x50_20_Obj_00> : Inport
  Bus Creator : BusCreator  Inputs=2  OutDataTypeStr=Bus: FUS_UINT8_RESERVED_ST
      settings: InheritFromInputs=off
  Bus Creator1 : BusCreator  Inputs=17  OutDataTypeStr=Bus: FUS_RADAR_OBJ_ST  NonVirtualBus=on
      settings: InheritFromInputs=off
  Bus Selector1 : BusSelector  OutputSignals=Obj_ObstacleProb,Obj_XPos_Stdev,Obj_YPos_Stdev,Obj_XVelRel_Stdev,Obj_XAccRel,Obj_ExstProb,Obj_YVelRel,Obj_XVelRel,Obj_XPos,Obj_YPos,Obj_ID,Obj_UpdateFlag,Obj_ValidFlag,Obj_MotionPattern,Obj_Type,Obj_MeasFlag
  Constant : Constant  Value=0  OutDataTypeStr=uint8
  Constant1 : Constant  Value=0  OutDataTypeStr=uint8
  Data Type Conversion : DataTypeConversion  OutDataTypeStr=uint16
  Data Type Conversion{1..5} (5 alike) : DataTypeConversion  OutDataTypeStr=uint8
  <OBJ_00> : Outport
  wires:
  Bus Selector1/10 -> Bus Creator1/10  "<Obj_YPos>"
  Constant1/1 -> Bus Creator/2
  Bus Selector1/8 -> Bus Creator1/8  "<Obj_XVelRel>"
  Bus Selector1/14 -> Data Type Conversion3/1  "<Obj_MotionPattern>"
  Bus Creator1/1 -> <OBJ_00>/1
  Bus Selector1/11 -> Data Type Conversion/1  "<Obj_ID>"
  Bus Selector1/16 -> Data Type Conversion5/1  "<Obj_MeasFlag>"
  Bus Selector1/2 -> Bus Creator1/2  "<Obj_XPos_Stdev>"
  Bus Selector1/6 -> Bus Creator1/6  "<Obj_ExstProb>"
  Bus Selector1/1 -> Bus Creator1/1  "<Obj_ObstacleProb>"
  Bus Selector1/15 -> Data Type Conversion4/1  "<Obj_Type>"
  Constant/1 -> Bus Creator/1
  Bus Selector1/13 -> Data Type Conversion2/1  "<Obj_ValidFlag>"
  Bus Selector1/9 -> Bus Creator1/9  "<Obj_XPos>"
  Bus Selector1/4 -> Bus Creator1/4  "<Obj_XVelRel_Stdev>"
  Bus Selector1/3 -> Bus Creator1/3  "<Obj_YPos_Stdev>"
  Bus Selector1/5 -> Bus Creator1/5  "<Obj_XAccRel>"
  Bus Selector1/7 -> Bus Creator1/7  "<Obj_YVelRel>"
  Bus Selector1/12 -> Data Type Conversion1/1  "<Obj_UpdateFlag>"
  <x50_20_Obj_00>/1 -> Bus Selector1/1
  Bus Creator/1 -> Bus Creator1/17
  Data Type Conversion/1 -> Bus Creator1/11  "obj_ID"
  Data Type Conversion1/1 -> Bus Creator1/12  "Obj_UpdateFlag"
  Data Type Conversion2/1 -> Bus Creator1/13
  Data Type Conversion3/1 -> Bus Creator1/14
  Data Type Conversion4/1 -> Bus Creator1/15
  Data Type Conversion5/1 -> Bus Creator1/16  "Obj_MeasFlag"

== system fusionAlg/FUSION /FUS_DataAdapter/RadarAdapter/Subsystem1 ==
  <x50_21_Obj_01> : Inport
  Bus Creator : BusCreator  Inputs=2  OutDataTypeStr=Bus: FUS_UINT8_RESERVED_ST
      settings: InheritFromInputs=off
  Bus Creator1 : BusCreator  Inputs=17  OutDataTypeStr=Bus: FUS_RADAR_OBJ_ST  NonVirtualBus=on
      settings: InheritFromInputs=off
  Bus Selector1 : BusSelector  OutputSignals=Obj_ObstacleProb,Obj_XPos_Stdev,Obj_YPos_Stdev,Obj_XVelRel_Stdev,Obj_XAccRel,Obj_ExstProb,Obj_YVelRel,Obj_XVelRel,Obj_XPos,Obj_YPos,Obj_ID,Obj_UpdateFlag,Obj_ValidFlag,Obj_MotionPattern,Obj_Type,Obj_MeasFlag
  Constant : Constant  Value=0  OutDataTypeStr=uint8
  Constant1 : Constant  Value=0  OutDataTypeStr=uint8
  Data Type Conversion : DataTypeConversion  OutDataTypeStr=uint16
  Data Type Conversion{1..5} (5 alike) : DataTypeConversion  OutDataTypeStr=uint8
  <OBJ_01> : Outport
  wires:
  Bus Selector1/10 -> Bus Creator1/10  "<Obj_YPos>"
  Constant1/1 -> Bus Creator/2
  Bus Selector1/8 -> Bus Creator1/8  "<Obj_XVelRel>"
  Bus Selector1/14 -> Data Type Conversion3/1  "<Obj_MotionPattern>"
  Bus Creator1/1 -> <OBJ_01>/1
  Bus Selector1/11 -> Data Type Conversion/1  "<Obj_ID>"
  Bus Selector1/16 -> Data Type Conversion5/1  "<Obj_MeasFlag>"
  Bus Selector1/2 -> Bus Creator1/2  "<Obj_XPos_Stdev>"
  Bus Selector1/6 -> Bus Creator1/6  "<Obj_ExstProb>"
  Bus Selector1/1 -> Bus Creator1/1  "<Obj_ObstacleProb>"
  Bus Selector1/15 -> Data Type Conversion4/1  "<Obj_Type>"
  Constant/1 -> Bus Creator/1
  Bus Selector1/13 -> Data Type Conversion2/1  "<Obj_ValidFlag>"
  Bus Selector1/9 -> Bus Creator1/9  "<Obj_XPos>"
  Bus Selector1/4 -> Bus Creator1/4  "<Obj_XVelRel_Stdev>"
  Bus Selector1/3 -> Bus Creator1/3  "<Obj_YPos_Stdev>"
  Bus Selector1/5 -> Bus Creator1/5  "<Obj_XAccRel>"
  Bus Selector1/7 -> Bus Creator1/7  "<Obj_YVelRel>"
  Bus Selector1/12 -> Data Type Conversion1/1  "<Obj_UpdateFlag>"
  <x50_21_Obj_01>/1 -> Bus Selector1/1
  Bus Creator/1 -> Bus Creator1/17
  Data Type Conversion/1 -> Bus Creator1/11
  Data Type Conversion1/1 -> Bus Creator1/12
  Data Type Conversion2/1 -> Bus Creator1/13
  Data Type Conversion3/1 -> Bus Creator1/14
  Data Type Conversion4/1 -> Bus Creator1/15
  Data Type Conversion5/1 -> Bus Creator1/16

== system fusionAlg/FUSION /FUS_DataAdapter/RadarAdapter/Subsystem10 ==
  <x5A_2A_Obj_10> : Inport
  Bus Creator : BusCreator  Inputs=2  OutDataTypeStr=Bus: FUS_UINT8_RESERVED_ST
      settings: InheritFromInputs=off
  Bus Creator1 : BusCreator  Inputs=17  OutDataTypeStr=Bus: FUS_RADAR_OBJ_ST  NonVirtualBus=on
      settings: InheritFromInputs=off
  Bus Selector1 : BusSelector  OutputSignals=Obj_ObstacleProb,Obj_XPos_Stdev,Obj_YPos_Stdev,Obj_XVelRel_Stdev,Obj_XAccRel,Obj_ExstProb,Obj_YVelRel,Obj_XVelRel,Obj_XPos,Obj_YPos,Obj_ID,Obj_UpdateFlag,Obj_ValidFlag,Obj_MotionPattern,Obj_Type,Obj_MeasFlag
  Constant : Constant  Value=0  OutDataTypeStr=uint8
  Constant1 : Constant  Value=0  OutDataTypeStr=uint8
  Data Type Conversion : DataTypeConversion  OutDataTypeStr=uint16
  Data Type Conversion{1..5} (5 alike) : DataTypeConversion  OutDataTypeStr=uint8
  <OBJ_10> : Outport
  wires:
  Bus Selector1/10 -> Bus Creator1/10  "<Obj_YPos>"
  Constant1/1 -> Bus Creator/2
  Bus Selector1/8 -> Bus Creator1/8  "<Obj_XVelRel>"
  Bus Selector1/14 -> Data Type Conversion3/1  "<Obj_MotionPattern>"
  Bus Creator1/1 -> <OBJ_10>/1
  Bus Selector1/11 -> Data Type Conversion/1  "<Obj_ID>"
  Bus Selector1/16 -> Data Type Conversion5/1  "<Obj_MeasFlag>"
  Bus Selector1/2 -> Bus Creator1/2  "<Obj_XPos_Stdev>"
  Bus Selector1/6 -> Bus Creator1/6  "<Obj_ExstProb>"
  Bus Selector1/1 -> Bus Creator1/1  "<Obj_ObstacleProb>"
  Bus Selector1/15 -> Data Type Conversion4/1  "<Obj_Type>"
  Constant/1 -> Bus Creator/1
  Bus Selector1/13 -> Data Type Conversion2/1  "<Obj_ValidFlag>"
  Bus Selector1/9 -> Bus Creator1/9  "<Obj_XPos>"
  Bus Selector1/4 -> Bus Creator1/4  "<Obj_XVelRel_Stdev>"
  Bus Selector1/3 -> Bus Creator1/3  "<Obj_YPos_Stdev>"
  Bus Selector1/5 -> Bus Creator1/5  "<Obj_XAccRel>"
  Bus Selector1/7 -> Bus Creator1/7  "<Obj_YVelRel>"
  Bus Selector1/12 -> Data Type Conversion1/1  "<Obj_UpdateFlag>"
  <x5A_2A_Obj_10>/1 -> Bus Selector1/1
  Bus Creator/1 -> Bus Creator1/17
  Data Type Conversion/1 -> Bus Creator1/11
  Data Type Conversion1/1 -> Bus Creator1/12
  Data Type Conversion2/1 -> Bus Creator1/13
  Data Type Conversion3/1 -> Bus Creator1/14
  Data Type Conversion4/1 -> Bus Creator1/15
  Data Type Conversion5/1 -> Bus Creator1/16

== system fusionAlg/FUSION /FUS_DataAdapter/RadarAdapter/Subsystem11 ==
  <x5B_2B_Obj_11> : Inport
  Bus Creator : BusCreator  Inputs=2  OutDataTypeStr=Bus: FUS_UINT8_RESERVED_ST
      settings: InheritFromInputs=off
  Bus Creator1 : BusCreator  Inputs=17  OutDataTypeStr=Bus: FUS_RADAR_OBJ_ST  NonVirtualBus=on
      settings: InheritFromInputs=off
  Bus Selector1 : BusSelector  OutputSignals=Obj_ObstacleProb,Obj_XPos_Stdev,Obj_YPos_Stdev,Obj_XVelRel_Stdev,Obj_XAccRel,Obj_ExstProb,Obj_YVelRel,Obj_XVelRel,Obj_XPos,Obj_YPos,Obj_ID,Obj_UpdateFlag,Obj_ValidFlag,Obj_MotionPattern,Obj_Type,Obj_MeasFlag
  Constant : Constant  Value=0  OutDataTypeStr=uint8
  Constant1 : Constant  Value=0  OutDataTypeStr=uint8
  Data Type Conversion : DataTypeConversion  OutDataTypeStr=uint16
  Data Type Conversion{1..5} (5 alike) : DataTypeConversion  OutDataTypeStr=uint8
  <OBJ_11> : Outport
  wires:
  Bus Selector1/10 -> Bus Creator1/10  "<Obj_YPos>"
  Constant1/1 -> Bus Creator/2
  Bus Selector1/8 -> Bus Creator1/8  "<Obj_XVelRel>"
  Bus Selector1/14 -> Data Type Conversion3/1  "<Obj_MotionPattern>"
  Bus Creator1/1 -> <OBJ_11>/1
  Bus Selector1/11 -> Data Type Conversion/1  "<Obj_ID>"
  Bus Selector1/16 -> Data Type Conversion5/1  "<Obj_MeasFlag>"
  Bus Selector1/2 -> Bus Creator1/2  "<Obj_XPos_Stdev>"
  Bus Selector1/6 -> Bus Creator1/6  "<Obj_ExstProb>"
  Bus Selector1/1 -> Bus Creator1/1  "<Obj_ObstacleProb>"
  Bus Selector1/15 -> Data Type Conversion4/1  "<Obj_Type>"
  Constant/1 -> Bus Creator/1
  Bus Selector1/13 -> Data Type Conversion2/1  "<Obj_ValidFlag>"
  Bus Selector1/9 -> Bus Creator1/9  "<Obj_XPos>"
  Bus Selector1/4 -> Bus Creator1/4  "<Obj_XVelRel_Stdev>"
  Bus Selector1/3 -> Bus Creator1/3  "<Obj_YPos_Stdev>"
  Bus Selector1/5 -> Bus Creator1/5  "<Obj_XAccRel>"
  Bus Selector1/7 -> Bus Creator1/7  "<Obj_YVelRel>"
  Bus Selector1/12 -> Data Type Conversion1/1  "<Obj_UpdateFlag>"
  <x5B_2B_Obj_11>/1 -> Bus Selector1/1
  Bus Creator/1 -> Bus Creator1/17
  Data Type Conversion/1 -> Bus Creator1/11
  Data Type Conversion1/1 -> Bus Creator1/12
  Data Type Conversion2/1 -> Bus Creator1/13
  Data Type Conversion3/1 -> Bus Creator1/14
  Data Type Conversion4/1 -> Bus Creator1/15
  Data Type Conversion5/1 -> Bus Creator1/16

== system fusionAlg/FUSION /FUS_DataAdapter/RadarAdapter/Subsystem12 ==
  <x5C_2C_Obj_12> : Inport
  Bus Creator : BusCreator  Inputs=2  OutDataTypeStr=Bus: FUS_UINT8_RESERVED_ST
      settings: InheritFromInputs=off
  Bus Creator1 : BusCreator  Inputs=17  OutDataTypeStr=Bus: FUS_RADAR_OBJ_ST  NonVirtualBus=on
      settings: InheritFromInputs=off
  Bus Selector1 : BusSelector  OutputSignals=Obj_ObstacleProb,Obj_XPos_Stdev,Obj_YPos_Stdev,Obj_XVelRel_Stdev,Obj_XAccRel,Obj_ExstProb,Obj_YVelRel,Obj_XVelRel,Obj_XPos,Obj_YPos,Obj_ID,Obj_UpdateFlag,Obj_ValidFlag,Obj_MotionPattern,Obj_Type,Obj_MeasFlag
  Constant : Constant  Value=0  OutDataTypeStr=uint8
  Constant1 : Constant  Value=0  OutDataTypeStr=uint8
  Data Type Conversion : DataTypeConversion  OutDataTypeStr=uint16
  Data Type Conversion{1..5} (5 alike) : DataTypeConversion  OutDataTypeStr=uint8
  <OBJ_12> : Outport
  wires:
  Bus Selector1/10 -> Bus Creator1/10  "<Obj_YPos>"
  Constant1/1 -> Bus Creator/2
  Bus Selector1/8 -> Bus Creator1/8  "<Obj_XVelRel>"
  Bus Selector1/14 -> Data Type Conversion3/1  "<Obj_MotionPattern>"
  Bus Creator1/1 -> <OBJ_12>/1
  Bus Selector1/11 -> Data Type Conversion/1  "<Obj_ID>"
  Bus Selector1/16 -> Data Type Conversion5/1  "<Obj_MeasFlag>"
  Bus Selector1/2 -> Bus Creator1/2  "<Obj_XPos_Stdev>"
  Bus Selector1/6 -> Bus Creator1/6  "<Obj_ExstProb>"
  Bus Selector1/1 -> Bus Creator1/1  "<Obj_ObstacleProb>"
  Bus Selector1/15 -> Data Type Conversion4/1  "<Obj_Type>"
  Constant/1 -> Bus Creator/1
  Bus Selector1/13 -> Data Type Conversion2/1  "<Obj_ValidFlag>"
  Bus Selector1/9 -> Bus Creator1/9  "<Obj_XPos>"
  Bus Selector1/4 -> Bus Creator1/4  "<Obj_XVelRel_Stdev>"
  Bus Selector1/3 -> Bus Creator1/3  "<Obj_YPos_Stdev>"
  Bus Selector1/5 -> Bus Creator1/5  "<Obj_XAccRel>"
  Bus Selector1/7 -> Bus Creator1/7  "<Obj_YVelRel>"
  Bus Selector1/12 -> Data Type Conversion1/1  "<Obj_UpdateFlag>"
  <x5C_2C_Obj_12>/1 -> Bus Selector1/1
  Bus Creator/1 -> Bus Creator1/17
  Data Type Conversion/1 -> Bus Creator1/11
  Data Type Conversion1/1 -> Bus Creator1/12
  Data Type Conversion2/1 -> Bus Creator1/13
  Data Type Conversion3/1 -> Bus Creator1/14
  Data Type Conversion4/1 -> Bus Creator1/15
  Data Type Conversion5/1 -> Bus Creator1/16

== system fusionAlg/FUSION /FUS_DataAdapter/RadarAdapter/Subsystem13 ==
  <x5D_2D_Obj_13> : Inport
  Bus Creator : BusCreator  Inputs=2  OutDataTypeStr=Bus: FUS_UINT8_RESERVED_ST
      settings: InheritFromInputs=off
  Bus Creator1 : BusCreator  Inputs=17  OutDataTypeStr=Bus: FUS_RADAR_OBJ_ST  NonVirtualBus=on
      settings: InheritFromInputs=off
  Bus Selector1 : BusSelector  OutputSignals=Obj_ObstacleProb,Obj_XPos_Stdev,Obj_YPos_Stdev,Obj_XVelRel_Stdev,Obj_XAccRel,Obj_ExstProb,Obj_YVelRel,Obj_XVelRel,Obj_XPos,Obj_YPos,Obj_ID,Obj_UpdateFlag,Obj_ValidFlag,Obj_MotionPattern,Obj_Type,Obj_MeasFlag
  Constant : Constant  Value=0  OutDataTypeStr=uint8
  Constant1 : Constant  Value=0  OutDataTypeStr=uint8
  Data Type Conversion : DataTypeConversion  OutDataTypeStr=uint16
  Data Type Conversion{1..5} (5 alike) : DataTypeConversion  OutDataTypeStr=uint8
  <OBJ_13> : Outport
  wires:
  Bus Selector1/10 -> Bus Creator1/10  "<Obj_YPos>"
  Constant1/1 -> Bus Creator/2
  Bus Selector1/8 -> Bus Creator1/8  "<Obj_XVelRel>"
  Bus Selector1/14 -> Data Type Conversion3/1  "<Obj_MotionPattern>"
  Bus Creator1/1 -> <OBJ_13>/1
  Bus Selector1/11 -> Data Type Conversion/1  "<Obj_ID>"
  Bus Selector1/16 -> Data Type Conversion5/1  "<Obj_MeasFlag>"
  Bus Selector1/2 -> Bus Creator1/2  "<Obj_XPos_Stdev>"
  Bus Selector1/6 -> Bus Creator1/6  "<Obj_ExstProb>"
  Bus Selector1/1 -> Bus Creator1/1  "<Obj_ObstacleProb>"
  Bus Selector1/15 -> Data Type Conversion4/1  "<Obj_Type>"
  Constant/1 -> Bus Creator/1
  Bus Selector1/13 -> Data Type Conversion2/1  "<Obj_ValidFlag>"
  Bus Selector1/9 -> Bus Creator1/9  "<Obj_XPos>"
  Bus Selector1/4 -> Bus Creator1/4  "<Obj_XVelRel_Stdev>"
  Bus Selector1/3 -> Bus Creator1/3  "<Obj_YPos_Stdev>"
  Bus Selector1/5 -> Bus Creator1/5  "<Obj_XAccRel>"
  Bus Selector1/7 -> Bus Creator1/7  "<Obj_YVelRel>"
  Bus Selector1/12 -> Data Type Conversion1/1  "<Obj_UpdateFlag>"
  <x5D_2D_Obj_13>/1 -> Bus Selector1/1
  Bus Creator/1 -> Bus Creator1/17
  Data Type Conversion/1 -> Bus Creator1/11
  Data Type Conversion1/1 -> Bus Creator1/12
  Data Type Conversion2/1 -> Bus Creator1/13
  Data Type Conversion3/1 -> Bus Creator1/14
  Data Type Conversion4/1 -> Bus Creator1/15
  Data Type Conversion5/1 -> Bus Creator1/16

== system fusionAlg/FUSION /FUS_DataAdapter/RadarAdapter/Subsystem14 ==
  <x66_36_Obj_22> : Inport
  Bus Creator : BusCreator  Inputs=2  OutDataTypeStr=Bus: FUS_UINT8_RESERVED_ST
      settings: InheritFromInputs=off
  Bus Creator1 : BusCreator  Inputs=17  OutDataTypeStr=Bus: FUS_RADAR_OBJ_ST  NonVirtualBus=on
      settings: InheritFromInputs=off
  Bus Selector1 : BusSelector  OutputSignals=Obj_ObstacleProb,Obj_XPos_Stdev,Obj_YPos_Stdev,Obj_XVelRel_Stdev,Obj_XAccRel,Obj_ExstProb,Obj_YVelRel,Obj_XVelRel,Obj_XPos,Obj_YPos,Obj_ID,Obj_UpdateFlag,Obj_ValidFlag,Obj_MotionPattern,Obj_Type,Obj_MeasFlag
  Constant : Constant  Value=0  OutDataTypeStr=uint8
  Constant1 : Constant  Value=0  OutDataTypeStr=uint8
  Data Type Conversion : DataTypeConversion  OutDataTypeStr=uint16
  Data Type Conversion{1..5} (5 alike) : DataTypeConversion  OutDataTypeStr=uint8
  <OBJ_22> : Outport
  wires:
  Bus Selector1/10 -> Bus Creator1/10  "<Obj_YPos>"
  Constant1/1 -> Bus Creator/2
  Bus Selector1/8 -> Bus Creator1/8  "<Obj_XVelRel>"
  Bus Selector1/14 -> Data Type Conversion3/1  "<Obj_MotionPattern>"
  Bus Creator1/1 -> <OBJ_22>/1
  Bus Selector1/11 -> Data Type Conversion/1  "<Obj_ID>"
  Bus Selector1/16 -> Data Type Conversion5/1  "<Obj_MeasFlag>"
  Bus Selector1/2 -> Bus Creator1/2  "<Obj_XPos_Stdev>"
  Bus Selector1/6 -> Bus Creator1/6  "<Obj_ExstProb>"
  Bus Selector1/1 -> Bus Creator1/1  "<Obj_ObstacleProb>"
  Bus Selector1/15 -> Data Type Conversion4/1  "<Obj_Type>"
  Constant/1 -> Bus Creator/1
  Bus Selector1/13 -> Data Type Conversion2/1  "<Obj_ValidFlag>"
  Bus Selector1/9 -> Bus Creator1/9  "<Obj_XPos>"
  Bus Selector1/4 -> Bus Creator1/4  "<Obj_XVelRel_Stdev>"
  Bus Selector1/3 -> Bus Creator1/3  "<Obj_YPos_Stdev>"
  Bus Selector1/5 -> Bus Creator1/5  "<Obj_XAccRel>"
  Bus Selector1/7 -> Bus Creator1/7  "<Obj_YVelRel>"
  Bus Selector1/12 -> Data Type Conversion1/1  "<Obj_UpdateFlag>"
  <x66_36_Obj_22>/1 -> Bus Selector1/1
  Bus Creator/1 -> Bus Creator1/17
  Data Type Conversion/1 -> Bus Creator1/11
  Data Type Conversion1/1 -> Bus Creator1/12
  Data Type Conversion2/1 -> Bus Creator1/13
  Data Type Conversion3/1 -> Bus Creator1/14
  Data Type Conversion4/1 -> Bus Creator1/15
  Data Type Conversion5/1 -> Bus Creator1/16
